simulink model "RobotController"  (R2017a)
settings: Solver=VariableStepAuto  StartTime=0.0  StopTime=200.0  RelTol=1e-3
settings Model: Creator=Carapinha  LastModifiedBy=Carapinha

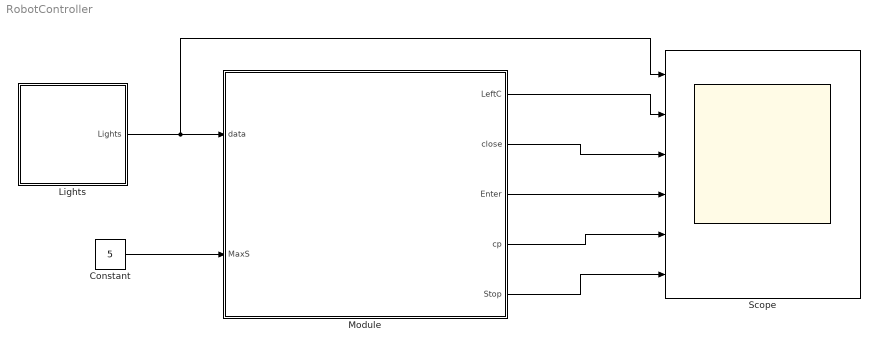
== system RobotController ==
  Constant : Constant  Value=5
  Lights : Stateflow chart  TreatAsAtomicUnit=on
  Module : Stateflow chart  TreatAsAtomicUnit=on
  Scope : Scope  NumInputPorts=6
  wires:
  Lights/1(Lights) -> Scope/1, Module/1(data)
  Module/1(LeftC) -> Scope/2
  Module/2(close) -> Scope/3
  Module/3(Enter) -> Scope/4
  Module/4(cp) -> Scope/5
  Module/5(Stop) -> Scope/6
  Constant/1 -> Module/2(MaxS)

== stateflow chart RobotController/Lights ==
  state Red
    entry:
    Lights = 0;
  state Green
    entry:
    Lights = 1;
  (default) -> Red
  Green -> Red : [after(0.7, sec)]
  Red -> Green : [after(0.7,sec)]
  data: Lights output

== stateflow chart RobotController/Module ==
  state Main
    state Robot [parallel]
      settings: executionOrder=1
      state move3
        entry:
        LeftC = 0;
        close = 0;
        Enter = 1;
        cp = 0;
        Stop = 0;
      state move1
        entry:
        LeftC = 1;
        close = 0;
        Enter = 0;
        cp = 0;
        Stop = 0;
      state move2
        entry:
        LeftC = 0;
        close = 1;
        Enter = 0;
        cp = 0;
        Stop = 0;
      state Accel
        entry:
        LeftC = 0;
        close = 0;
        Enter = 1;
        cp = 0;
        Stop = 0;
        speed = acc(10);
      state Decel
        entry:
        LeftC = 0;
        close = 0;
        Enter = 0;
        cp = 1;
        Stop = 0;
        speed = acc(-5);
      state Wait
        entry:
        LeftC = 0;
        close = 0;
        Enter = 0;
        cp = 0;
        Stop = 1;
      move3 -> move1 : [after(0.3,sec)]
      (default) -> move1
      move1 -> move2 : [after(0.3,sec)]
      move2 -> move3 [order 1] : [Permission == 1]
      Accel -> move3 : [speed == MaxS]
      move2 -> Decel [order 2] : [after(0.3,sec)]
      Decel -> Accel [order 1] : [Permission == 1]
      Decel -> Wait [order 2] : [speed == 0]
      Wait -> Accel [order 1] : [Permission == 1]
      Wait -> Wait [order 2] : [Permission == 0]
    state Controller [parallel]
      settings: executionOrder=2
      state RobotState
      state Green
        entry:
        Permission = 1;
      state RobotState3
      state Red
        entry:
        Permission = 0;
      RobotState3 -> RobotState : [LeftC == 1]
      (default) -> RobotState
      Green -> RobotState3 : [after(1.1,sec)]
      RobotState -> (junction 79) : [close == 1 || Stop == 1]
      (junction 79) -> Green [order 1] : [data == 1]
      (junction 79) -> Red [order 2] : [data == 0]
      Red -> RobotState
  (default) -> Main
  data: data input; LeftC output; close output; Enter output; cp output; Stop output; MaxS input; Permission local; speed local
